simulink model "Copy_of_BEV_projekat"  (R2018a)
settings: Solver=VariableStepAuto  StartTime=0.0  StopTime=1000  FixedStep=.1  MaxStep=1e-3  RelTol=1e-3  EnableMultiTasking=on
PostLoadFcn:
  | addpath('ImagesBEV')
  | 
  | BEVDir = pwd;
  | 
  | cd ..\;
  | SimulinkDir = pwd;
  | addpath(SimulinkDir);
  | 
  | cd(BEVDir);
StopFcn:
  | MotorNetTorque = results.Motor.MotorNetTorque_Nm_;
  | SOC = results.Battery.SOC___;
  | BatteryPowerAtTerminals = results.Battery.BatteryPowerAtTerminals_W_;
  | VehicleSpeed = results.Glider.Velocity_kmh_;
  | 
  | figure
  | scatter(VehicleSpeed.get.Data(:),MotorNetTorque.get.Data(:),'.')
  | grid on
  | box on
  | title('Motor Torque vs. Vehicle Speed')
  | xlabel('Vehicle Speed, V (kmh)')
  | ylabel('Motor Torque, Tm (Nm)')
  | 
  | figure
  | scatter(VehicleSpeed.get.Data(:),BatteryPowerAtTerminals.get.Data(:))
  | grid on
  | box on
  | title('Battery Power vs. Vehicle Speed')
  | xlabel('Vehicle Speed, (kmh)')
  | ylabel('Power, (kW)')
  | 
  | figure
  | plot(SOC.get.Time(:),SOC.get.Data(:))
  | grid on
  | box on
  | title('SOC vs. Time')
  | xlabel('Time (s)')
  | ylabel('SOC (%)')
  | 
  | clear MotorNetTorque SOC BatteryPowerAtTerminals VehicleSpeed ;
model workspace (MAT data in the model file):
  AccessoryLoad = 600
  C_ref = 600
  DrCycles.C505 = [0 1 2 3 4 5 6 7 8 9 10 11 ... (1012 elements, 506x2)]
  DrCycles.FTP = [0 1 2 3 4 5 6 7 8 9 10 11 ... (4956 elements, 2478x2)]
  DrCycles.UDDS = [0 1 2 3 4 5 6 7 8 9 10 11 ... (2746 elements, 1373x2)]
  DrCycles.HWFET = [0 1 2 3 4 5 6 7 8 9 10 11 ... (1532 elements, 766x2)]
  DrCycles.US06 = [0 1 2 3 4 5 6 7 8 9 10 11 ... (1194 elements, 597x2)]
  DrCycles.US06City = [0 1 2 3 4 5 6 7 8 9 10 11 ... (466 elements, 233x2)]
  DrCycles.US06Hwy = [0 1 2 3 4 5 6 7 8 9 10 11 ... (742 elements, 371x2)]
  K = 1.04716227018
  Kc_ref = 0.12
  Ki_ref = 0.01
  Kw_ref = 1.2e-05
  MDL.MotorModel.kc = 0.0452374100719
  MDL.MotorModel.ki = 0.0166666666667
  MDL.MotorModel.kw = 5.06640055941e-05
  MDL.MotorModel.C = 628.29736211
  MDL.MotorModel.MaxTrqOut = 500
  MDL.MotorModel.MaxPwrOut = 100000
  MDL.DrivelineModel.C0 = 600
  MDL.DrivelineModel.C1 = 0.012
  MDL.DrivelineModel.C2 = 4.9e-07
  MDL.DrivelineModel.G = 3.55
  MDL.DrivelineModel.Spinloss = 6
  MDL.DrivelineModel.Ftr_max = 5000
  MDL.DriverModel.Kp = 350
  MDL.DriverModel.Ki = 0
  MDL.DriverModel.Kd = 0
  MDL.DriverModel.BrakeGain = 100
  MDL.DriverModel.Ftr_Max = 5000
  MDL.DriverModel.Ptr_Max = 100000
  MDL.BrakeSys.MaxBrakeForce = 10000
  MDL.BrakeSys.RegenFraction = 0.55
  T_max = 500
  T_ref = 300
  TimeHWFET = 765
  TimeUDDS = 1372
  TimeUS06 = 596
  aeroDragCoeff = 0.38
  airDensity = 1.23
  energyCapacity = 12.6
  frontArea = 2.1
  gravity = 9.81
  inclinationAngle = 0
  inertialMassVeh = 2392
  initialSOC = 0.95
  internalResistance = 0.1
  massVeh = 2300
  openCircuitVoltage = 340
  rollingResistCoeff = 0.01
  w_max = 524
  w_ref = 834
  wheelRadius = 0.34
undefined symbols (not defined in the file): drag_koeficijent, kapac_bat, magnitude, Maks_mom_mot, Maks_snag_mot, otp_bat, poc_SOC
libraries: simulink x6, drivingcycle_lib x1
CloseFcn:
  | rmpath(SimulinkDir);
  | rmpath('ImagesBEV')
  | clear BEVDir SimulinkDir;
settings Model: Creator=David  LastModifiedBy=Goran Vujnovic
settings DataIOCC: ExternalInput=DrCycles.US06  LoadExternalInput=on  SaveFormat=Array
settings OptimizationCC: ExpressionDepthLimit=2147483647  LifeSpan=inf
settings DebuggingCC: UnderspecifiedInitializationDetection=Classic  MergeDetectMultiDrivingBlocksExec=none  SolverPrmCheckMsg=warning  FcnCallInpInsideContextMsg=warning  StateNameClashWarn=warning  SFUnexpectedBacktrackingDiag=warning  SFNoUnconditionalDefaultTransitionDiag=warning  SFExecutionAtInitializationDiag=none
settings HardwareCC: ProdBitPerPointer=32  ProdBitPerSizeT=32  ProdBitPerPtrDiffT=32  ProdLargestAtomicFloat=None  ProdIntDivRoundTo=Undefined  ProdEndianess=Unspecified  ProdWordSize=32  ProdHWDeviceType=32-bit Generic
settings ModelReferenceCC: PropagateSignalLabelsOutOfModel=off
settings CodeAppCC: StateflowObjectComments=on
settings GRTTargetCC: TargetLangStandard=C89/C90 (ANSI)  GeneratePreprocessorConditionals=Disable all  CombineOutputUpdateFcns=off  GRTInterface=on
settings ConfigComp: CovMetricSettings=dw  CovHtmlReporting=on  CovSaveCumulativeToWorkspaceVar=on  CovSaveSingleToWorkspaceVar=on  CovExternalEMLEnable=off  CovSFcnEnable=off

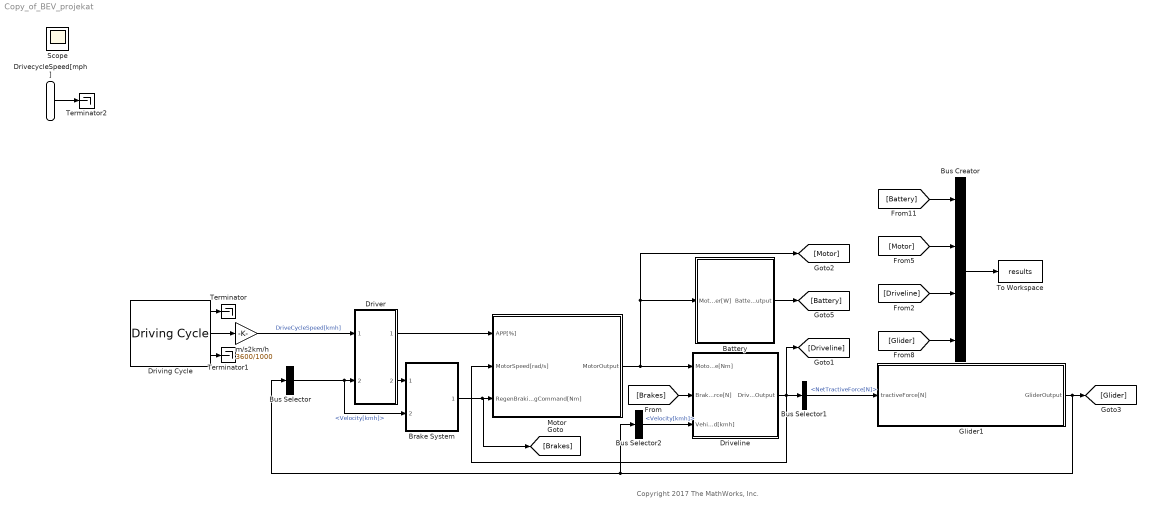
== system Copy_of_BEV_projekat ==
  note: Copyright 2017 The MathWorks, Inc.
  DrivecycleSpeed[mph] : Inport
  Battery : Subsystem
      mask Display: image('battery.jpg');
  Brake System : Subsystem
      mask Display: image('brakes.jpg');
  Bus Creator : BusCreator  Inputs=4
  Bus Selector : BusSelector  OutputSignals=Velocity[kmh]
  Bus Selector1 : BusSelector  OutputSignals=NetTractiveForce[N]
  Bus Selector2 : BusSelector  OutputSignals=Velocity[kmh]
  Driveline : Subsystem
      mask Display: image('driveline.jpg');
  Driver : Subsystem  AncestorBlock=Driver_Glider_Library/Driver
      mask Display: image('DriverPic.jpg');
  Driving Cycle : drivingcycle_lib/Driving Cycle  CycleName=ArtUrban  CycleRepeatsForever=on
      settings: SourceProductName=Driving Cycle Blockset
  Glider1 : Subsystem  AncestorBlock=Driver_Glider_Library/Glider
      mask Display: image('VehiclePic.jpg');
  Motor : Subsystem
      mask Display: image('motor.jpg');
  Terminator : Terminator
  Terminator1 : Terminator
  Terminator2 : Terminator
  To Workspace : ToWorkspace  VariableName=results  SaveFormat=Timeseries  SampleTime=-1
  m/s2km/h : Gain  Gain=3600/1000
  Scope : Scope
  wires:
  Driver/1(APP[%]) -> Motor/1(APP[%])
  Bus Creator/1 -> To Workspace/1
  Driver/2(BPP[%]) -> Brake System/1(BPP[%])
  [Brakes] -> Driveline/2(BrakeForce[N])
  Brake System/1(BrakeOutput) -> [Brakes], Motor/3(RegenBrakingCommand[Nm])
  [Driveline] -> Bus Creator/3
  Driveline/1(DrivelineOutput) -> Bus Selector1/1, Motor/2(MotorSpeed[rad/s]), [Driveline]
  [Motor] -> Bus Creator/2
  Motor/1(MotorOutput) -> [Motor], Battery/1(MotorPower[W]), Driveline/1(MotorTorque[Nm])
  [Glider] -> Bus Creator/4
  Glider1/1(GliderOutput) -> [Glider], Bus Selector/1, Bus Selector2/1
  Bus Selector/1 -> Brake System/2(VehicleSpeed[kmh]), Driver/2(VehicleSpeed[mph])  "<Velocity[kmh]>"
  Bus Selector2/1 -> Driveline/3(VehicleSpeed[kmh])  "<Velocity[kmh]>"
  [Battery] -> Bus Creator/1
  Battery/1(BatteryOutput) -> [Battery]
  Bus Selector1/1 -> Glider1/1(tractiveForce[N])  "<NetTractiveForce[N]>"
  Driving Cycle/3 -> Terminator1/1
  Driving Cycle/1 -> Terminator/1
  Driving Cycle/2 -> m/s2km/h/1
  DrivecycleSpeed[mph]/1 -> Terminator2/1
  m/s2km/h/1 -> Driver/1(DriveCycleSpeed[mph])  "DriveCycleSpeed[kmh]"

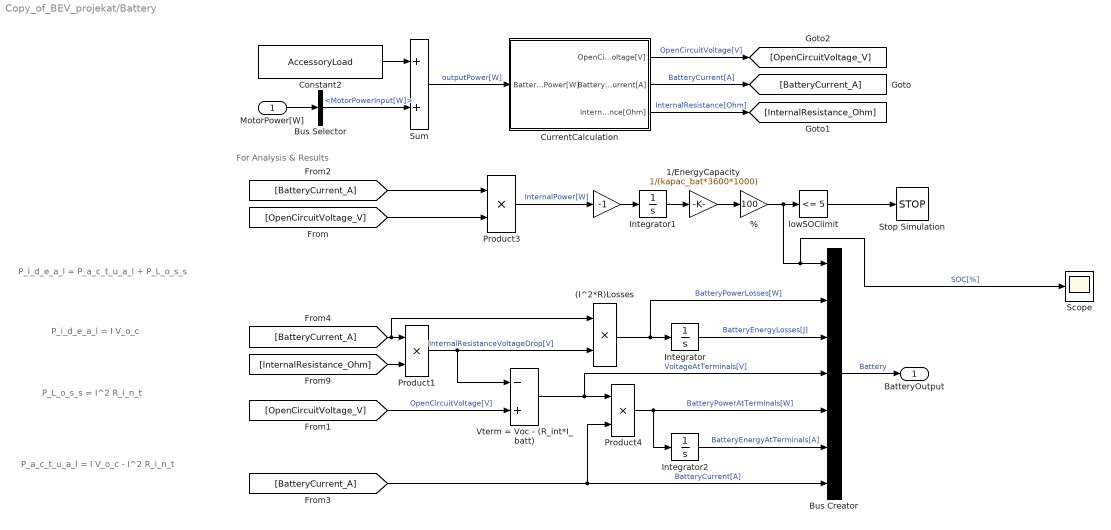
== system Copy_of_BEV_projekat/Battery ==
  note: For Analysis & Results
  note: P_i_d_e_a_l = I V_o_c
  note: P_i_d_e_a_l = P_a_c_t_u_a_l + P_L_o_s_s
  note: P_L_o_s_s = I^2 R_i_n_t
  note: P_a_c_t_u_a_l = I V_o_c - I^2 R_i_n_t
  MotorPower[W] : Inport
  " " : Gain  Gain=-1
  % : Gain  Gain=100
  (I^2*R)Losses : Product  RndMeth=Zero
  1/EnergyCapacity : Gain  Gain=1/(kapac_bat*3600*1000)
  Bus Creator : BusCreator  Inputs=7
  Bus Selector : BusSelector  OutputSignals=MotorPowerInput[W]
  Constant2 : Constant  Value=AccessoryLoad
  CurrentCalculation : Subsystem
  Integrator : Integrator  ZeroCross=off
  Integrator1 : Integrator  InitialCondition=kapac_bat*3600*1000*poc_SOC  ZeroCross=off
  Integrator2 : Integrator
  Product1 : Product  RndMeth=Zero
  Product3 : Product  RndMeth=Zero
  Product4 : Product  RndMeth=Zero
  Scope : Scope
  Stop Simulation : Stop
  Sum : Sum
  Vterm = Voc - (R_int*I_batt) : Sum  Inputs=-+
  lowSOClimit : simulink/Logic and Bit Operations/Compare To Constant  relop=<=  const=5  OutDataTypeStr=boolean
  BatteryOutput : Outport
  wires:
  Product1/1 -> (I^2*R)Losses/2, Vterm = Voc - (R_int*I_batt)/1  "InternalResistanceVoltageDrop[V]"
  (I^2*R)Losses/1 -> Bus Creator/2, Integrator/1  "BatteryPowerLosses[W]"
  Integrator/1 -> Bus Creator/3  "BatteryEnergyLosses[J]"
  Product3/1 -> " "/1  "InternalPower[W]"
  Integrator1/1 -> 1/EnergyCapacity/1
  Constant2/1 -> Sum/1
  Bus Creator/1 -> BatteryOutput/1  "Battery"
  1/EnergyCapacity/1 -> %/1
  MotorPower[W]/1 -> Bus Selector/1
  Sum/1 -> CurrentCalculation/1(BatteryPower[W])  "outputPower[W]"
  " "/1 -> Integrator1/1
  Bus Selector/1 -> Sum/2  "<MotorPowerInput[W]>"
  [OpenCircuitVoltage_V] -> Product3/2
  CurrentCalculation/1(OpenCircuitVoltage[V]) -> [OpenCircuitVoltage_V]  "OpenCircuitVoltage[V]"
  [OpenCircuitVoltage_V] -> Vterm = Voc - (R_int*I_batt)/2  "OpenCircuitVoltage[V]"
  [BatteryCurrent_A] -> Product3/1
  [BatteryCurrent_A] -> Bus Creator/7, Product4/2  "BatteryCurrent[A]"
  [BatteryCurrent_A] -> (I^2*R)Losses/1, Product1/1
  Vterm = Voc - (R_int*I_batt)/1 -> Bus Creator/4, Product4/1  "VoltageAtTerminals[V]"
  CurrentCalculation/2(BatteryCurrent[A]) -> [BatteryCurrent_A]  "BatteryCurrent[A]"
  CurrentCalculation/3(InternalResistance[Ohm]) -> [InternalResistance_Ohm]  "InternalResistance[Ohm]"
  [InternalResistance_Ohm] -> Product1/2
  Product4/1 -> Bus Creator/5, Integrator2/1  "BatteryPowerAtTerminals[W]"
  Integrator2/1 -> Bus Creator/6  "BatteryEnergyAtTerminals[A]"
  %/1 -> lowSOClimit/1, Scope/1, Bus Creator/1  "SOC[%]"
  lowSOClimit/1 -> Stop Simulation/1

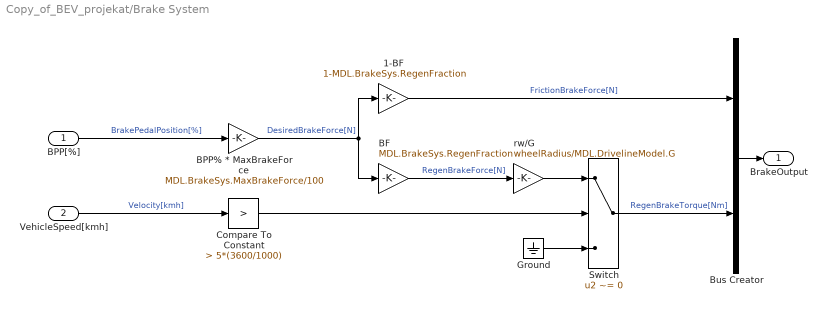
== system Copy_of_BEV_projekat/Brake System ==
  BPP[%] : Inport
  VehicleSpeed[kmh] : Inport  Port=2
  1-BF : Gain  Gain=1-MDL.BrakeSys.RegenFraction
  BF : Gain  Gain=MDL.BrakeSys.RegenFraction
  BPP% * MaxBrakeForce : Gain  Gain=MDL.BrakeSys.MaxBrakeForce/100
  Bus Creator : BusCreator  Inputs=2
  Compare To Constant : simulink/Logic and Bit Operations/Compare To Constant  relop=>  const=5*(3600/1000)  OutDataTypeStr=boolean
  Ground : Ground
  Switch : Switch  Criteria=u2 ~= 0
  rw/G : Gain  Gain=wheelRadius/MDL.DrivelineModel.G
  BrakeOutput : Outport
  wires:
  Bus Creator/1 -> BrakeOutput/1
  BPP[%]/1 -> BPP% * MaxBrakeForce/1  "BrakePedalPosition[%]"
  BPP% * MaxBrakeForce/1 -> BF/1, 1-BF/1  "DesiredBrakeForce[N]"
  BF/1 -> rw/G/1  "RegenBrakeForce[N]"
  1-BF/1 -> Bus Creator/1  "FrictionBrakeForce[N]"
  rw/G/1 -> Switch/1
  VehicleSpeed[kmh]/1 -> Compare To Constant/1  "Velocity[kmh]"
  Ground/1 -> Switch/3
  Switch/1 -> Bus Creator/2  "RegenBrakeTorque[Nm]"
  Compare To Constant/1 -> Switch/2

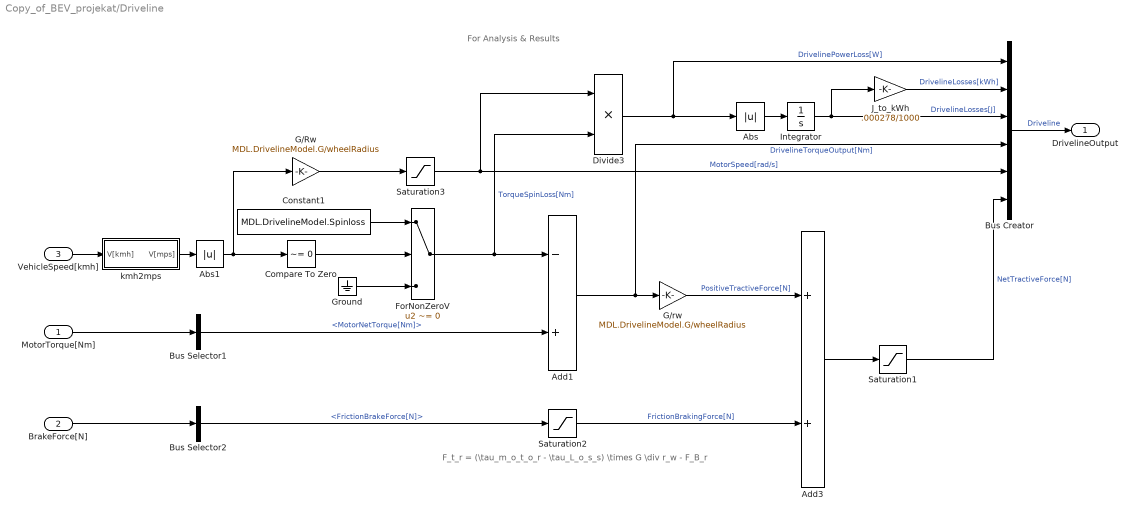
== system Copy_of_BEV_projekat/Driveline ==
  note: For Analysis & Results
  note: F_t_r = (\tau_m_o_t_o_r - \tau_L_o_s_s) \times G \div r_w - F_B_r
  MotorTorque[Nm] : Inport
  BrakeForce[N] : Inport  Port=2
  VehicleSpeed[kmh] : Inport  Port=3
  Abs : Abs  ZeroCross=off
  Abs1 : Abs  ZeroCross=off
  Add1 : Sum  Inputs=-+
  Add3 : Sum
  Bus Creator : BusCreator  Inputs=6
  Bus Selector1 : BusSelector  OutputSignals=MotorNetTorque[Nm]
  Bus Selector2 : BusSelector  OutputSignals=FrictionBrakeForce[N]
  Compare To Zero : simulink/Logic and Bit Operations/Compare To Zero  relop=~=  OutDataTypeStr=boolean
  Constant1 : Constant  Value=MDL.DrivelineModel.Spinloss
  Divide3 : Product  Inputs=**
  ForNonZeroV : Switch  Criteria=u2 ~= 0  ZeroCross=off
  G/Rw : Gain  Gain=MDL.DrivelineModel.G/wheelRadius
  G/rw : Gain  Gain=MDL.DrivelineModel.G/wheelRadius
  Ground : Ground
  Integrator : Integrator  ZeroCross=off
  J_to_kWh : Gain  Gain=.000278/1000
  Saturation1 : Saturate  UpperLimit=5000  LowerLimit=-10000  ZeroCross=off
  Saturation2 : Saturate  UpperLimit=0  LowerLimit=-10000  ZeroCross=off
  Saturation3 : Saturate  UpperLimit=inf  LowerLimit=0.00001  ZeroCross=off
  kmh2mps : Subsystem
  DrivelineOutput : Outport
  wires:
  G/rw/1 -> Add3/1  "PositiveTractiveForce[N]"
  Add3/1 -> Saturation1/1
  Abs/1 -> Integrator/1
  BrakeForce[N]/1 -> Bus Selector2/1
  Saturation2/1 -> Add3/2  "FrictionBrakingForce[N]"
  MotorTorque[Nm]/1 -> Bus Selector1/1
  G/Rw/1 -> Saturation3/1
  VehicleSpeed[kmh]/1 -> kmh2mps/1(V[kmh])
  ForNonZeroV/1 -> Divide3/2, Add1/1  "TorqueSpinLoss[Nm]"
  Add1/1 -> Bus Creator/4, G/rw/1  "DrivelineTorqueOutput[Nm]"
  Saturation3/1 -> Divide3/1, Bus Creator/5  "MotorSpeed[rad/s]"
  Divide3/1 -> Bus Creator/1, Abs/1  "DrivelinePowerLoss[W]"
  Saturation1/1 -> Bus Creator/6  "NetTractiveForce[N]"
  Abs1/1 -> Compare To Zero/1, G/Rw/1
  Bus Selector2/1 -> Saturation2/1  "<FrictionBrakeForce[N]>"
  J_to_kWh/1 -> Bus Creator/2  "DrivelineLosses[kWh]"
  Ground/1 -> ForNonZeroV/3
  Constant1/1 -> ForNonZeroV/1
  Bus Creator/1 -> DrivelineOutput/1  "Driveline"
  Integrator/1 -> J_to_kWh/1, Bus Creator/3  "DrivelineLosses[J]"
  Bus Selector1/1 -> Add1/2  "<MotorNetTorque[Nm]>"
  Compare To Zero/1 -> ForNonZeroV/2
  kmh2mps/1(V[mps]) -> Abs1/1

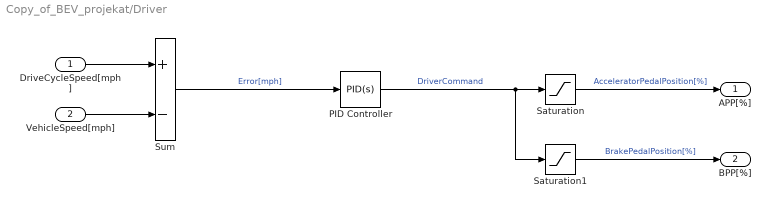
== system Copy_of_BEV_projekat/Driver ==
  DriveCycleSpeed[mph] : Inport
  VehicleSpeed[mph] : Inport  Port=2
  PID Controller : simulink/Continuous/PID Controller  Controller=PID  TimeDomain=Continuous-time  SampleTime=-1  IntegratorMethod=Forward Euler  FilterMethod=Forward Euler  Form=Parallel  UseFilter=on  ControllerParametersSource=internal  P=250  I=1  D=0  N=100  InitialConditionSource=internal  InitialConditionForIntegrator=0  InitialConditionForFilter=0  ExternalReset=none  LimitOutput=off  UpperSaturationLimit=inf  LowerSaturationLimit=-inf  LinearizeAsGain=on  AntiWindupMode=none  Kb=1  TrackingMode=off  Kt=1  PParamMin=[]  PParamMax=[]  IParamMin=[]  IParamMax=[]  DParamMin=[]  DParamMax=[]  NParamMin=[]  NParamMax=[]  KbParamMin=[]  KbParamMax=[]  KtParamMin=[]  KtParamMax=[]  POutMin=[]  POutMax=[]  IOutMin=[]  IOutMax=[]  DOutMin=[]  DOutMax=[]  NOutMin=[]  NOutMax=[]  KbOutMin=[]  KbOutMax=[]  KtOutMin=[]  KtOutMax=[]  IntegratorOutMin=[]  IntegratorOutMax=[]  FilterOutMin=[]  FilterOutMax=[]  SumOutMin=[]  SumOutMax=[]  SumI1OutMin=[]  SumI1OutMax=[]  SumI2OutMin=[]  SumI2OutMax=[]  SumI3OutMin=[]  SumI3OutMax=[]  SumDOutMin=[]  SumDOutMax=[]  SaturationOutMin=[]  SaturationOutMax=[]  IntegratorContinuousStateAttributes=''  IntegratorStateMustResolveToSignalObject=off  IntegratorRTWStateStorageClass=Auto  FilterContinuousStateAttributes=''  FilterStateMustResolveToSignalObject=off  FilterRTWStateStorageClass=Auto  DifferentiatorICPrevScaledInput=0  DifferentiatorOutMin=[]  DifferentiatorOutMax=[]  InitialConditionSetting=State (most efficient)  FilterDiffOutCoefMin=[]  FilterDiffOutCoefMax=[]  SumDenOutMin=[]  SumDenOutMax=[]  SumNumOutMin=[]  SumNumOutMax=[]  ReciprocalOutMin=[]  ReciprocalOutMax=[]  DivideOutMin=[]  DivideOutMax=[]  TunerSelectOption=Transfer Function Based (PID Tuner App)
  Saturation : Saturate  UpperLimit=100  LowerLimit=0  ZeroCross=off
  Saturation1 : Saturate  UpperLimit=0  LowerLimit=-100  ZeroCross=off
  Sum : Sum  Inputs=+-
  APP[%] : Outport
  BPP[%] : Outport  Port=2
  wires:
  DriveCycleSpeed[mph]/1 -> Sum/1
  Saturation/1 -> APP[%]/1  "AcceleratorPedalPosition[%]"
  PID Controller/1 -> Saturation1/1, Saturation/1  "DriverCommand"
  Saturation1/1 -> BPP[%]/1  "BrakePedalPosition[%]"
  Sum/1 -> PID Controller/1  "Error[mph]"
  VehicleSpeed[mph]/1 -> Sum/2

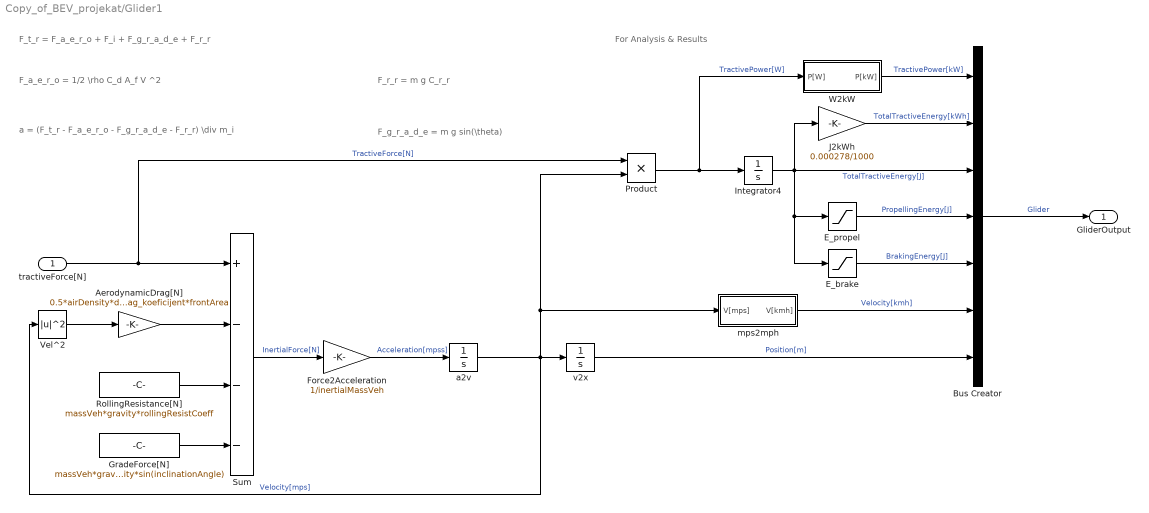
== system Copy_of_BEV_projekat/Glider1 ==
  note: F_t_r = F_a_e_r_o + F_i + F_g_r_a_d_e + F_r_r
  note: a = (F_t_r - F_a_e_r_o - F_g_r_a_d_e - F_r_r) \div m_i
  note: F_r_r = m g C_r_r
  note: For Analysis & Results
  note: F_a_e_r_o = 1/2 \rho C_d A_f V ^2
  note: F_g_r_a_d_e = m g sin(\theta)
  tractiveForce[N] : Inport
  AerodynamicDrag[N] : Gain  Gain=0.5*airDensity*drag_koeficijent*frontArea
      settings: AttributesFormatString=%<Gain>
  Bus Creator : BusCreator  Inputs=7
  E_brake : Saturate  UpperLimit=0  LowerLimit=-inf
  E_propel : Saturate  UpperLimit=inf  LowerLimit=0
  Force2Acceleration : Gain  Gain=1/inertialMassVeh
      settings: AttributesFormatString=%<Gain>
  GradeForce[N] : Constant  Value=massVeh*gravity*sin(inclinationAngle)
      settings: AttributesFormatString=%<Value>
  Integrator4 : Integrator
  J2kWh : Gain  Gain=0.000278/1000
  Product : Product
  RollingResistance[N] : Constant  Value=massVeh*gravity*rollingResistCoeff
      settings: AttributesFormatString=%<Value>
  Sum : Sum  Inputs=+---
  Vel^2 : Math  Operator=magnitude^2  SaturateOnIntegerOverflow=on
  W2kW : Subsystem
  a2v : Integrator
  mps2mph : Subsystem
  v2x : Integrator
  GliderOutput : Outport
  wires:
  J2kWh/1 -> Bus Creator/2  "TotalTractiveEnergy[kWh]"
  Sum/1 -> Force2Acceleration/1  "InertialForce[N]"
  mps2mph/1(V[kmh]) -> Bus Creator/6  "Velocity[kmh]"
  E_propel/1 -> Bus Creator/4  "PropellingEnergy[J]"
  W2kW/1(P[kW]) -> Bus Creator/1  "TractivePower[kW]"
  Vel^2/1 -> AerodynamicDrag[N]/1
  Integrator4/1 -> J2kWh/1, Bus Creator/3, E_brake/1, E_propel/1  "TotalTractiveEnergy[J]"
  Force2Acceleration/1 -> a2v/1  "Acceleration[mpss]"
  E_brake/1 -> Bus Creator/5  "BrakingEnergy[J]"
  RollingResistance[N]/1 -> Sum/3
  GradeForce[N]/1 -> Sum/4
  AerodynamicDrag[N]/1 -> Sum/2
  v2x/1 -> Bus Creator/7  "Position[m]"
  a2v/1 -> v2x/1, Vel^2/1, mps2mph/1(V[mps]), Product/2  "Velocity[mps]"
  tractiveForce[N]/1 -> Product/1, Sum/1  "TractiveForce[N]"
  Product/1 -> W2kW/1(P[W]), Integrator4/1  "TractivePower[W]"
  Bus Creator/1 -> GliderOutput/1  "Glider"

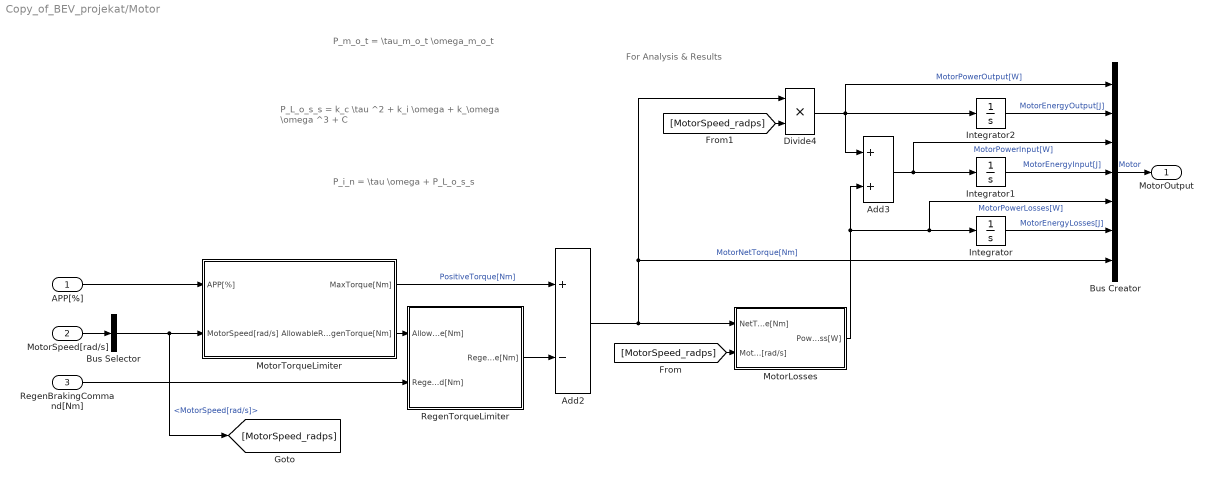
== system Copy_of_BEV_projekat/Motor ==
  note: P_i_n = \tau \omega + P_L_o_s_s
  note: For Analysis & Results
  note: P_L_o_s_s = k_c \tau ^2 + k_i \omega + k_\omega \omega ^3 + C
  note: P_m_o_t = \tau_m_o_t \omega_m_o_t
  APP[%] : Inport
  MotorSpeed[rad/s] : Inport  Port=2
  RegenBrakingCommand[Nm] : Inport  Port=3
  Add2 : Sum  Inputs=+-
  Add3 : Sum
  Bus Creator : BusCreator  Inputs=7
  Bus Selector : BusSelector  OutputSignals=MotorSpeed[rad/s]
  Divide4 : Product  Inputs=**
  Integrator : Integrator  ZeroCross=off
  Integrator1 : Integrator  ZeroCross=off
  Integrator2 : Integrator  ZeroCross=off
  MotorLosses : Subsystem
  MotorTorqueLimiter : Subsystem
  RegenTorqueLimiter : Subsystem
  MotorOutput : Outport
  wires:
  Add3/1 -> Bus Creator/3, Integrator1/1  "MotorPowerInput[W]"
  Divide4/1 -> Bus Creator/1, Add3/1, Integrator2/1  "MotorPowerOutput[W]"
  [MotorSpeed_radps] -> Divide4/2
  Integrator1/1 -> Bus Creator/4  "MotorEnergyInput[J]"
  Integrator2/1 -> Bus Creator/2  "MotorEnergyOutput[J]"
  Add2/1 -> MotorLosses/1(NetTorque[Nm]), Divide4/1, Bus Creator/7  "MotorNetTorque[Nm]"
  MotorTorqueLimiter/1(MaxTorque[Nm]) -> Add2/1  "PositiveTorque[Nm]"
  APP[%]/1 -> MotorTorqueLimiter/1(APP[%])
  MotorLosses/1(PowerLoss[W]) -> Bus Creator/5, Integrator/1, Add3/2  "MotorPowerLosses[W]"
  RegenBrakingCommand[Nm]/1 -> RegenTorqueLimiter/2(RegenBrakeCommand[Nm])
  MotorTorqueLimiter/2(AllowableRegenTorque[Nm]) -> RegenTorqueLimiter/1(AllowableRegenTorque[Nm])
  RegenTorqueLimiter/1(RegenTorque[Nm]) -> Add2/2
  [MotorSpeed_radps] -> MotorLosses/2(MotorSpeed[rad/s])
  Bus Creator/1 -> MotorOutput/1  "Motor"
  Integrator/1 -> Bus Creator/6  "MotorEnergyLosses[J]"
  MotorSpeed[rad/s]/1 -> Bus Selector/1
  Bus Selector/1 -> MotorTorqueLimiter/2(MotorSpeed[rad/s]), [MotorSpeed_radps]  "<MotorSpeed[rad/s]>"

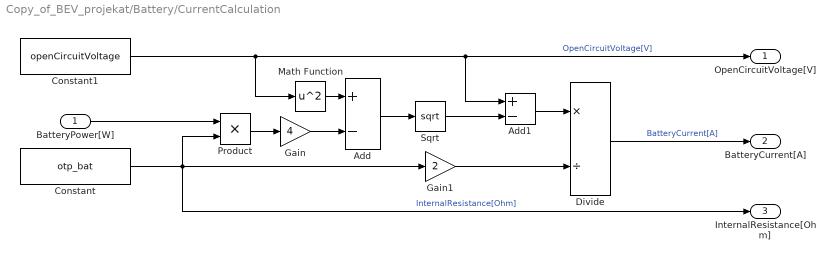
== system Copy_of_BEV_projekat/Battery/CurrentCalculation ==
  BatteryPower[W] : Inport
  Add : Sum  Inputs=+-
  Add1 : Sum  Inputs=+-
  Constant : Constant  Value=otp_bat
  Constant1 : Constant  Value=openCircuitVoltage
  Divide : Product  Inputs=*/
  Gain : Gain  Gain=4
  Gain1 : Gain  Gain=2
  Math Function : Math  Operator=square  SaturateOnIntegerOverflow=on
  Product : Product  RndMeth=Zero
  Sqrt : Sqrt  SaturateOnIntegerOverflow=on
  OpenCircuitVoltage[V] : Outport
  BatteryCurrent[A] : Outport  Port=2
  InternalResistance[Ohm] : Outport  Port=3
  wires:
  BatteryPower[W]/1 -> Product/1
  Constant/1 -> InternalResistance[Ohm]/1, Gain1/1, Product/2  "InternalResistance[Ohm]"
  Product/1 -> Gain/1
  Constant1/1 -> Math Function/1, OpenCircuitVoltage[V]/1, Add1/1  "OpenCircuitVoltage[V]"
  Math Function/1 -> Add/1
  Gain/1 -> Add/2
  Sqrt/1 -> Add1/2
  Add/1 -> Sqrt/1
  Add1/1 -> Divide/1
  Gain1/1 -> Divide/2
  Divide/1 -> BatteryCurrent[A]/1  "BatteryCurrent[A]"

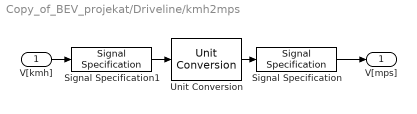
== system Copy_of_BEV_projekat/Driveline/kmh2mps ==
  V[kmh] : Inport
  Signal Specification : SignalSpecification  Unit=m/s
  Signal Specification1 : SignalSpecification  Unit=km/h
  Unit Conversion : UnitConversion
  V[mps] : Outport
  wires:
  V[kmh]/1 -> Signal Specification1/1
  Unit Conversion/1 -> Signal Specification/1
  Signal Specification1/1 -> Unit Conversion/1
  Signal Specification/1 -> V[mps]/1

== system Copy_of_BEV_projekat/Glider1/W2kW ==
  P[W] : Inport
  Signal Specification : SignalSpecification  Unit=kW
  Signal Specification1 : SignalSpecification  Unit=W
  Unit Conversion : UnitConversion
  P[kW] : Outport
  wires:
  Signal Specification/1 -> P[kW]/1
  Signal Specification1/1 -> Unit Conversion/1
  Unit Conversion/1 -> Signal Specification/1
  P[W]/1 -> Signal Specification1/1

== system Copy_of_BEV_projekat/Glider1/mps2mph ==
  V[mps] : Inport
  Signal Specification : SignalSpecification  Unit=km/h
  Signal Specification1 : SignalSpecification  Unit=m/s
  Unit Conversion : UnitConversion
  V[kmh] : Outport
  wires:
  V[mps]/1 -> Signal Specification1/1
  Unit Conversion/1 -> Signal Specification/1
  Signal Specification1/1 -> Unit Conversion/1
  Signal Specification/1 -> V[kmh]/1

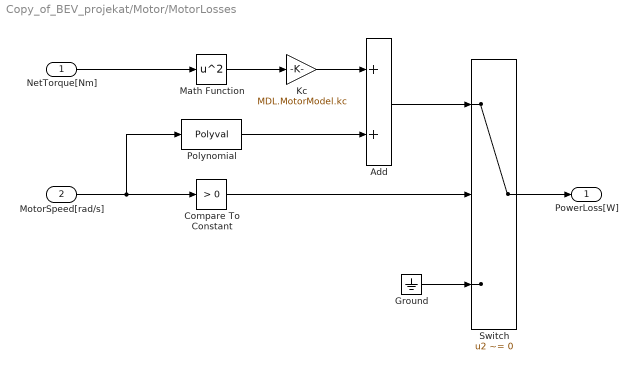
== system Copy_of_BEV_projekat/Motor/MotorLosses ==
  NetTorque[Nm] : Inport
  MotorSpeed[rad/s] : Inport  Port=2
  Add : Sum
  Compare To Constant : simulink/Logic and Bit Operations/Compare To Constant  relop=>  const=0  OutDataTypeStr=boolean
  Ground : Ground
  Kc : Gain  Gain=MDL.MotorModel.kc
  Math Function : Math  Operator=square  SaturateOnIntegerOverflow=on
  Polynomial : Polyval  Coefs=[MDL.MotorModel.kw , 0 ,MDL.MotorModel.ki, MDL.MotorModel.C]
  Switch : Switch  Criteria=u2 ~= 0  ZeroCross=off
  PowerLoss[W] : Outport
  wires:
  NetTorque[Nm]/1 -> Math Function/1
  Math Function/1 -> Kc/1
  Kc/1 -> Add/1
  MotorSpeed[rad/s]/1 -> Polynomial/1, Compare To Constant/1
  Ground/1 -> Switch/3
  Switch/1 -> PowerLoss[W]/1
  Polynomial/1 -> Add/2
  Add/1 -> Switch/1
  Compare To Constant/1 -> Switch/2

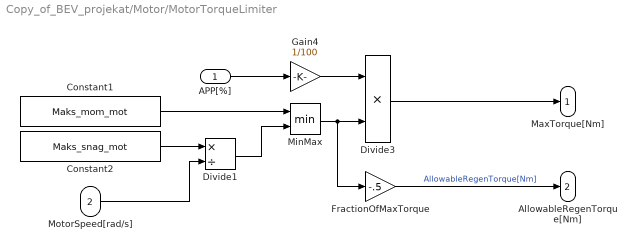
== system Copy_of_BEV_projekat/Motor/MotorTorqueLimiter ==
  APP[%] : Inport
  MotorSpeed[rad/s] : Inport  Port=2
  Constant1 : Constant  Value=Maks_mom_mot
  Constant2 : Constant  Value=Maks_snag_mot
  Divide1 : Product  Inputs=*/
  Divide3 : Product  Inputs=**
  FractionOfMaxTorque : Gain  Gain=-.5
  Gain4 : Gain  Gain=1/100
  MinMax : MinMax  Inputs=2
  MaxTorque[Nm] : Outport
  AllowableRegenTorque[Nm] : Outport  Port=2
  wires:
  Constant1/1 -> MinMax/1
  MinMax/1 -> FractionOfMaxTorque/1, Divide3/2
  Gain4/1 -> Divide3/1
  APP[%]/1 -> Gain4/1
  Divide3/1 -> MaxTorque[Nm]/1
  Constant2/1 -> Divide1/1
  Divide1/1 -> MinMax/2
  MotorSpeed[rad/s]/1 -> Divide1/2
  FractionOfMaxTorque/1 -> AllowableRegenTorque[Nm]/1  "AllowableRegenTorque[Nm]"

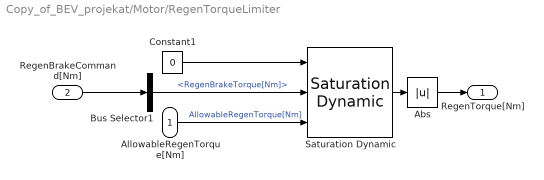
== system Copy_of_BEV_projekat/Motor/RegenTorqueLimiter ==
  AllowableRegenTorque[Nm] : Inport
  RegenBrakeCommand[Nm] : Inport  Port=2
  Abs : Abs
  Bus Selector1 : BusSelector  OutputSignals=RegenBrakeTorque[Nm]
  Constant1 : Constant  Value=0
  Saturation Dynamic : simulink/Discontinuities/Saturation Dynamic  OutMin=[]  OutMax=[]  OutDataTypeStr=Inherit: Same as second input  OutDataType=fixdt(1, 16)  OutScaling=2^-10  DoSatur=off
  RegenTorque[Nm] : Outport
  wires:
  AllowableRegenTorque[Nm]/1 -> Saturation Dynamic/3  "AllowableRegenTorque[Nm]"
  Constant1/1 -> Saturation Dynamic/1
  Bus Selector1/1 -> Saturation Dynamic/2  "<RegenBrakeTorque[Nm]>"
  RegenBrakeCommand[Nm]/1 -> Bus Selector1/1
  Saturation Dynamic/1 -> Abs/1
  Abs/1 -> RegenTorque[Nm]/1
